simulink model "PWPF"  (R2023a)
settings: Solver=daessc  StartTime=0.0  StopTime=10.0  RelTol=1e-5
settings Model: Creator=cnsl  LastModifiedBy=cnsl
settings SolverCC: ZeroCrossAlgorithm=Adaptive
settings DebuggingCC: AlgebraicLoopMsg=none

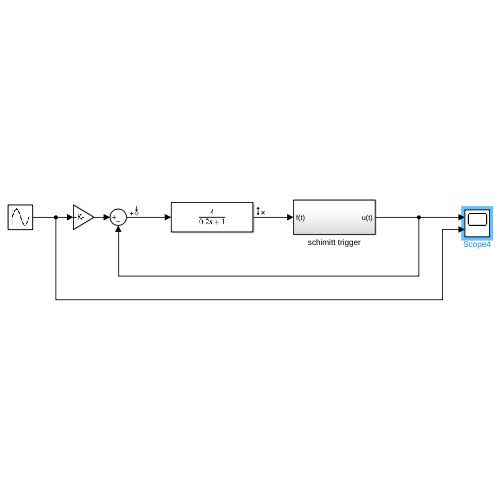
[thumbnail: Simulink's stored preview of the top-level diagram]
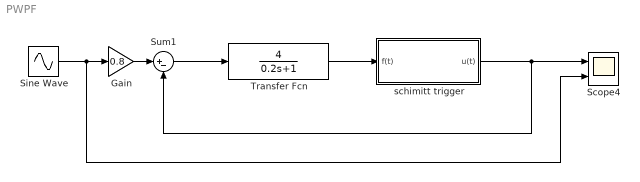
== system PWPF ==
  Gain : Gain  Gain=0.8
  Scope4 : Scope  NumInputPorts=2
  Sine Wave : Sin  Frequency=0.1*2*pi  SampleTime=0
  Sum1 : Sum  Inputs=|+-
  Transfer Fcn : TransferFcn  Numerator=[4]  Denominator=[0.2 1]
  schimitt trigger : Subsystem
  wires:
  Sum1/1 -> Transfer Fcn/1
  schimitt trigger/1(u(t)) -> Sum1/2, Scope4/1
  Transfer Fcn/1 -> schimitt trigger/1(f(t))
  Sine Wave/1 -> Scope4/2, Gain/1
  Gain/1 -> Sum1/1

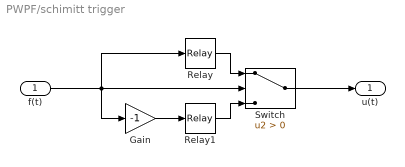
== system PWPF/schimitt trigger ==
  f(t) : Inport
  Gain : Gain  Gain=-1
  Relay : Relay  OnSwitchValue=0.5  OffSwitchValue=0.15
  Relay1 : Relay  OnSwitchValue=0.5  OffSwitchValue=0.15  OnOutputValue=-1
  Switch : Switch  Criteria=u2 > Threshold  SaturateOnIntegerOverflow=off  InputSameDT=off
  u(t) : Outport
  wires:
  f(t)/1 -> Relay/1, Gain/1, Switch/2
  Relay1/1 -> Switch/3
  Gain/1 -> Relay1/1
  Relay/1 -> Switch/1
  Switch/1 -> u(t)/1
